simulink library "groundStation001_cl"  (R2020a)
settings: Solver=VariableStepAuto  StartTime=0.0  StopTime=10.0  RelTol=1e-3
values from neighbouring files (symbols this model uses):
  D = sum(normalVecMat'.*relVelGnd',2)    [oceanForceFunct.m]
undefined symbols (not defined in the file or in its folder): gndStn, numNodes
libraries: vrlib x2, tethersMoment_cl x2, thrAttachPtKinematics_ul x2, simulink x1, tether000_cl x1, bouyancyCalculator_ul x1, oceanForceCalculator_ul x1, sixDoFDynamicsEuler_ul x1
settings Model: Creator=Erin B  LastModifiedBy=jcreed2
settings DataIOCC: ReturnWorkspaceOutputs=off
settings DebuggingCC: ArithmeticOperatorsInVariantConditions=warning
settings SFSimCC: CustomCodeUndefinedFunction=UseInterfaceOnly

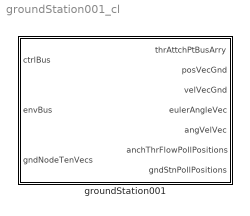
== system groundStation001_cl ==
  groundStation001 : Subsystem  VariantControl=VSS_groundStation_groundStation001  mask{gs=gndStn, numNodes=numNodes}
      mask prompts: gs "Ground Station"; numNodes "Number of anchor tether nodes"
      mask init:
      | groundStation001_init

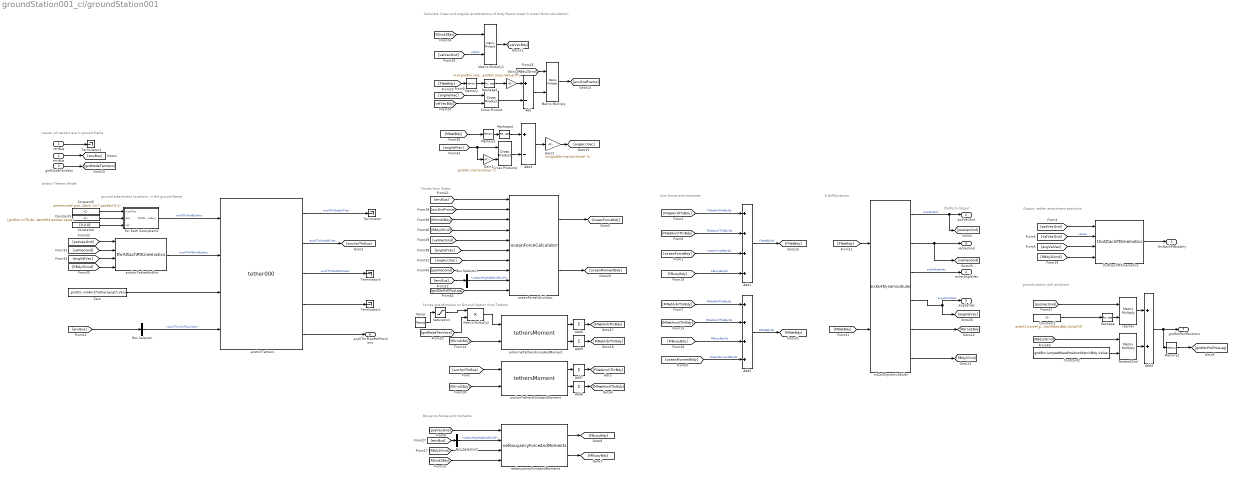
== system groundStation001_cl/groundStation001 ==
  note: ground station poll positions
  note: Bouyancy forces and moments
  note: Calculate linear and angular accelerations of body frame
      | (used in ocean force calculation)
  note: ground attachment locations, in the ground frame
  note: Platform Output
  note: Anchor Tethers Model
  note: Forces and Moments on Ground Station from Tethers
  note: Output: tether attachment positions
  note: Inputs, all vectors are in ground frame
  note: Sum forces and moments
  note: 6 DoFDynamics
  note: Forces from Ocean
  ctrlBus : Inport  OutDataTypeStr=Bus: gndStnCtrlBus
  envBus : Inport  Port=2  OutDataTypeStr=Bus: envBus
  gndNodeTenVecs : Inport  Port=3
  Add : Sum  Inputs=+-
  Add1 : Sum  Inputs=++++
  Add2 : Sum  Inputs=++++
  Add3 : Sum  Inputs=+-
  Add4 : Sum
  Add{6..9} (4 alike) : Sum  Inputs=+  CollapseMode=Specified dimension  CollapseDim=2
  Bus Selector : BusSelector  OutputSignals=anchThrLinkFlowVecs
  Bus Selector1 : BusSelector  OutputSignals=oceanHeightAtGndStnLM
  Bus Selector2 : BusSelector  OutputSignals=oceanHeightAtGndStnLM
  Constant1 : Constant  Value=ones(1,numel(gndStn.lumpedMassPositionMatrixBdy.Value)/3)
  Constant2 : Constant  Value=gndStn.lumpedMassPositionMatrixBdy.Value
  Constant3 : Constant  Value=[gndStn.inrThrAttchPt1.posVec.Value,gndStn.inrThrAttchPt2.posVec.Value,gndStn.inrThrAttchPt3.posVec.Value]
  Constant4 : Constant  Value=[0,0,0]'
  Constant5 : Constant  Value=ones(numel(gndStn.struct('OCT.thrAttch','inr').posVec)/3,1)
  Cross Product : vrlib/Utilities/Cross Product
  Cross Product4 : vrlib/Utilities/Cross Product
  For Each Subsystem1 : Subsystem  TreatAsAtomicUnit=on
  Gain1 : Gain  Gain=inv([gndStn.mass.Value,0,0;0,gndStn.mass.Value,0;0,0,gndStn.mass.Value])  Multiplication=Matrix(K*u)
  Gain2 : Gain  Gain=inv(gndStn.inertia.Value)  Multiplication=Matrix(K*u)
  Gain3 : Gain  Gain=gndStn.inertia.Value  Multiplication=Matrix(K*u)
  Matrix Multiply : Product  Multiplication=Matrix(*)
  Matrix Multiply1 : Product  Multiplication=Matrix(*)
  Matrix Multiply2 : Product
  Memory : Memory
  Memory1 : Memory
  Memory2 : Memory  InitialCondition=gndStn.lumpedMassPositionMatrixBdy.Value
  Ramp : simulink/Sources/Ramp  slope=.0025  start=400  InitialOutput=0
  Reshape : Reshape  OutputDimensionality=Row vector (2-D)
  Reshape1 : Reshape  OutputDimensionality=Column vector (2-D)
  Reshape4 : Reshape  OutputDimensionality=Column vector (2-D)
  Rotate2Gnd : Product  Multiplication=Matrix(*)
  Saturation : Saturate
  Terminator{,1..2,5} (4 alike) : Terminator
  Zero : Constant  Value=gndStn.initAnchTetherLength.Value  OutDataTypeStr=Inherit: Inherit via back propagation
  airborneTethersForceAndMoment : tethersMoment_cl/tethersMoment  arms=gs.struct('OCT.thrAttch','kit')
  anchorTetherEndPnt : thrAttachPtKinematics_ul/thrAttachPtKinematics  atchPts=gs.struct('OCT.thrAttch','plt')
  anchorTethers : tether000_cl/tether000  VariantControl=VSS_tethers_tether000  LabelModeActiveChoice=twoNodeTether  numNodes=numNodes  thrStructure=gs.anchThrs.struct('OCT.tether')  fluidDensity=env.water.density.Value  gravity=env.gravAccel.Value
  anchorTethersForceAndMoment : tethersMoment_cl/tethersMoment  arms=gs.struct('OCT.thrAttch','plt')
  netbouyancyForceAndMoments : bouyancyCalculator_ul/netbouyancyForceAndMoments  SystemSampleTime=-1  Latency=0  AutoFrameSizeCalculation=off
  oceanForceCalculator : oceanForceCalculator_ul/oceanForceCalculator  Cdx=gndStn.cdX.Value  Cdy=gndStn.cdY.Value  Cdz=gndStn.cdZ.Value  Cax=gndStn.aMX.Value  Cay=gndStn.aMY.Value  Caz=gndStn.aMZ.Value  V=gndStn.volume.Value/(numel(gndStn.lumpedMassPositionMatrixBdy.Value)/3)
  repmat : Product  Multiplication=Matrix(*)
  sixDoFDynamicsEuler : sixDoFDynamicsEuler_ul/sixDoFDynamicsEuler  VariantControl=(default)  M=gndStn.mass.Value  J=gndStn.inertia.Value  initPos=gndStn.initPosVecGnd.Value  initVel=gndStn.initVelVecBdy.Value  initEulAngs=gndStn.initEulAng.Value  initAngVel=gndStn.initAngVelVec.Value
  thrAttachPtKinematics : thrAttachPtKinematics_ul/thrAttachPtKinematics  atchPts=gs.struct('OCT.thrAttch','kit')
  thrAttchPtBusArry : Outport  VectorParamsAs1DForOutWhenUnconnected=off
  posVecGnd : Outport  Port=2  VectorParamsAs1DForOutWhenUnconnected=off
  velVecGnd : Outport  Port=3  VectorParamsAs1DForOutWhenUnconnected=off
  eulerAngleVec : Outport  Port=4  VectorParamsAs1DForOutWhenUnconnected=off
  angVelVec : Outport  Port=5  VectorParamsAs1DForOutWhenUnconnected=off
  anchThrFlowPollPositions : Outport  Port=6  VectorParamsAs1DForOutWhenUnconnected=off
  gndStnPollPositions : Outport  Port=7  VectorParamsAs1DForOutWhenUnconnected=off
  wires:
  [MBuoyBdy] -> Add2/3  "MBuoyBdyGs"
  [FNetBdy] -> sixDoFDynamicsEuler/1
  anchorTethers/3 -> Terminator5/1  "anchThrNodePosVecs"
  Add1/1 -> [FNetBdy]  "FNetBdyGs"
  anchorTethers/2 -> [anchorThrBus]  "anchThrNodeNFVec"
  anchorTethers/1 -> Terminator/1  "anchThrNode1FVec"
  sixDoFDynamicsEuler/3 -> eulerAngleVec/1  "eulerAngleVec"
  anchorTetherEndPnt/1 -> anchorTethers/2  "anchThrPltfrmBusArry"
  sixDoFDynamicsEuler/1 -> [posVecGnd], posVecGnd/1  "posVecGnd"
  [RGrnd2Bdy] -> anchorTethersForceAndMoment/2
  [MNetBdy] -> sixDoFDynamicsEuler/2
  [posVecGnd] -> netbouyancyForceAndMoments/1
  [posVecGnd] -> anchorTetherEndPnt/1
  [angVelVec] -> anchorTetherEndPnt/3
  [RBdy2Grnd] -> anchorTetherEndPnt/4
  [velVecGnd] -> anchorTetherEndPnt/2
  anchorTethersForceAndMoment/1 -> Add7/1
  anchorTethersForceAndMoment/2 -> Add8/1
  Add7/1 -> [FNetAnchThrBdy]
  Add8/1 -> [MNetAnchThrBdy]
  [velVecGnd] -> thrAttachPtKinematics/2  "velVec"
  [RBdy2Grnd] -> thrAttachPtKinematics/4
  [angVelVec] -> thrAttachPtKinematics/3
  [posVecGnd] -> thrAttachPtKinematics/1
  thrAttachPtKinematics/1 -> thrAttchPtBusArry/1
  gndNodeTenVecs/1 -> [gndNodeTenVecs]
  Add2/1 -> [MNetBdy]  "MNetBdyGs"
  ctrlBus/1 -> Terminator1/1
  envBus/1 -> [envBus]
  [oceanForceBdy] -> Add1/3  "oceanForceBdyGs"
  [RGrnd2Bdy] -> airborneTethersForceAndMoment/2
  Add9/1 -> [MNetAibrThrBdy]
  Add6/1 -> [FNetAirbThrBdy]
  airborneTethersForceAndMoment/1 -> Add6/1
  airborneTethersForceAndMoment/2 -> Add9/1
  [anchorThrBus] -> anchorTethersForceAndMoment/1
  [FNetAirbThrBdy] -> Add1/1  "FNetAirbThrBdyGs"
  [FNetAnchThrBdy] -> Add1/2  "FNetAnchThrBdyGs"
  [MNetAibrThrBdy] -> Add2/1  "MNetAibrThrBdyGs"
  [MNetAnchThrBdy] -> Add2/2  "MNetAnchThrBdyGs"
  [FBuoyBdy] -> Add1/4  "FBuoyBdyGs"
  [envBus] -> oceanForceCalculator/1
  oceanForceCalculator/1 -> [oceanForceBdy]
  sixDoFDynamicsEuler/2 -> [velVecGnd], velVecGnd/1
  sixDoFDynamicsEuler/4 -> [angVelVec], angVelVec/1  "angularVelVec"
  sixDoFDynamicsEuler/5 -> [RGrnd2Bdy]
  sixDoFDynamicsEuler/6 -> [RBdy2Grnd]
  anchorTethers/4 -> Terminator2/1
  netbouyancyForceAndMoments/2 -> [MBuoyBdy]
  netbouyancyForceAndMoments/1 -> [FBuoyBdy]
  [RGrnd2Bdy] -> netbouyancyForceAndMoments/4
  [RBdy2Grnd] -> netbouyancyForceAndMoments/3
  [angVelVec] -> Cross Product/1
  [velVecBdy] -> Cross Product/2
  Cross Product/1 -> Add/2
  [FNetBdy] -> Memory/1
  Reshape1/1 -> Gain1/1
  Gain1/1 -> Add/1
  Add/1 -> Matrix Multiply/2
  [RBdy2Grnd] -> Matrix Multiply/1
  [velVecGnd] -> Matrix Multiply1/2  "velVec"
  [RGrnd2Bdy] -> Matrix Multiply1/1
  Matrix Multiply1/1 -> [velVecBdy]
  Matrix Multiply/1 -> [accGndFrame]
  [angVelVec] -> Cross Product4/1, Gain3/1
  [MNetBdy] -> Memory1/1
  Cross Product4/1 -> Add3/2
  Add3/1 -> Gain2/1
  Reshape4/1 -> Add3/1
  Gain3/1 -> Cross Product4/2
  Gain2/1 -> [angAccVec]
  [accGndFrame] -> oceanForceCalculator/2
  oceanForceCalculator/2 -> [oceanMomentBdy]
  [oceanMomentBdy] -> Add2/4  "OceanMomentBdyGs"
  [velVecGnd] -> oceanForceCalculator/5
  [angAccVec] -> oceanForceCalculator/7
  [angVelVec] -> oceanForceCalculator/6
  [RGrnd2Bdy] -> oceanForceCalculator/3
  [RBdy2Grnd] -> oceanForceCalculator/4
  repmat/1 -> Add4/1
  [RBdy2Grnd] -> Rotate2Gnd/1
  Rotate2Gnd/1 -> Add4/2
  Constant2/1 -> Rotate2Gnd/2
  Constant1/1 -> Reshape/1
  [posVecGnd] -> repmat/1
  Zero/1 -> anchorTethers/3
  For Each Subsystem1/1(thrAttchPtBusArry) -> anchorTethers/1  "anchThrGndBusArry"
  [envBus] -> Bus Selector/1
  Bus Selector/1 -> anchorTethers/4  "<anchThrLinkFlowVecs>"
  Reshape/1 -> repmat/2
  Memory/1 -> Reshape1/1
  Memory1/1 -> Reshape4/1
  [posVecGnd] -> oceanForceCalculator/8
  Constant5/1 -> For Each Subsystem1/1(numPos)
  Constant4/1 -> For Each Subsystem1/3(vel)
  Constant3/1 -> For Each Subsystem1/2(pos)
  anchorTethers/5 -> anchThrFlowPollPositions/1
  [envBus] -> Bus Selector1/1
  Bus Selector1/1 -> oceanForceCalculator/9  "<oceanHeightAtGndStnLM>"
  Bus Selector2/1 -> netbouyancyForceAndMoments/2  "<oceanHeightAtGndStnLM>"
  [envBus] -> Bus Selector2/1
  Add4/1 -> Memory2/1, gndStnPollPositions/1
  Memory2/1 -> [gndStnPollPosLag]
  [gndStnPollPosLag] -> oceanForceCalculator/10
  [gndNodeTenVecs] -> Matrix Multiply2/2
  Matrix Multiply2/1 -> airborneTethersForceAndMoment/1
  Ramp/1 -> Saturation/1
  Saturation/1 -> Matrix Multiply2/1

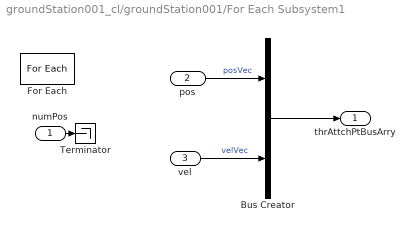
== system groundStation001_cl/groundStation001/For Each Subsystem1 ==
  numPos : Inport  Partition=on  PartitionDimension=1  PartitionWidth=1  PartitionOffset=0
  pos : Inport  Port=2  Partition=on  PartitionDimension=2  PartitionWidth=1  PartitionOffset=0
  vel : Inport  Port=3
  Bus Creator : BusCreator  Inputs=2  OutDataTypeStr=Bus: thrAttachPtKinematicsBus  NonVirtualBus=on
  For Each : ForEach  DisableCoverage=on
  Terminator : Terminator
  thrAttchPtBusArry : Outport  ConcatenationDimension=1  VectorParamsAs1DForOutWhenUnconnected=off
  wires:
  pos/1 -> Bus Creator/1  "posVec"
  Bus Creator/1 -> thrAttchPtBusArry/1
  vel/1 -> Bus Creator/2  "velVec"
  numPos/1 -> Terminator/1
